simulink model "formationControl"  (R2021b)
settings: Solver=FixedStepAuto  StartTime=0.0  StopTime=20  FixedStep=0.01  RelTol=1e-3
values from neighbouring files (symbols this model uses):
  optimalPath = cat(1,optimalPath,invPathTemp)    [CompareBruteForce.m]    (also in main2.m; main3.m; main5.m; main6.m)
  startPoint1 = [currentX;currentY;atan2(optimalPath(i,2)+.5-currentY,optimalPath(i,1)+.5-currentX)]    [main2.m]    (also in main3.m = [currentX1;currentY1;atan2(optimalPath(i,2)+.5-currentY1,opt; main5.m = [currentX1;currentY1;theta_x1]; main6.m = [currentX1;currentY1;atan2(optimalPath(i,2)+.5-currentY1,opt; main7.m = [currentX1;currentY1;theta_x1])
  startPoint2 = [currentX2;currentY2;currentTeta2]    [main3.m]    (also in main5.m; main6.m; main7.m; main8.m = [currentX2;currentY2;theta_x1])
  startPoint3 = [currentX3;currentY3;currentTeta3]    [main3.m]    (also in main5.m; main6.m; main7.m; main8.m = [currentX3;currentY3;theta_x1])
  targetPoint1 = [optimalPath(1,1)+.5,optimalPath(1,2)+.5]    [main2.m]    (also in main3.m; main5.m; main6.m; main7.m)
  theta = toDegree(x(3))    [CalcHeadingEval.m]    (also in DynamicWindowApproachSample.m; main3.m = atan2(dy,dx); main5.m = atan2(dy,dx); main6.m = atan2(dy,dx))
  v = 3    [mTSPandFormation.m]    (also in main3.m = sqrt(vx.^2+vy.^2); main5.m = sqrt(vx.^2+vy.^2); main6.m = sqrt(vx.^2+vy.^2); main7.m = sqrt(vx.^2+vy.^2))
  vw_dt = [0.04;0]    [main3.m]    (also in main5.m; main6.m; main7.m; main8.m)
  w = edgew(p(j,k),p(j,k+1))    [CompareBruteForce.m]    (also in main3.m = dtheta ./ gradient(t_temp); main5.m = dtheta ./ gradient(t_temp); main6.m = dtheta ./ gradient(t_temp); main7.m = dtheta ./ gradient(t_temp))
settings Model: Creator=laptop  LastModifiedBy=SPKT2021
settings DataIOCC: ReturnWorkspaceOutputs=off

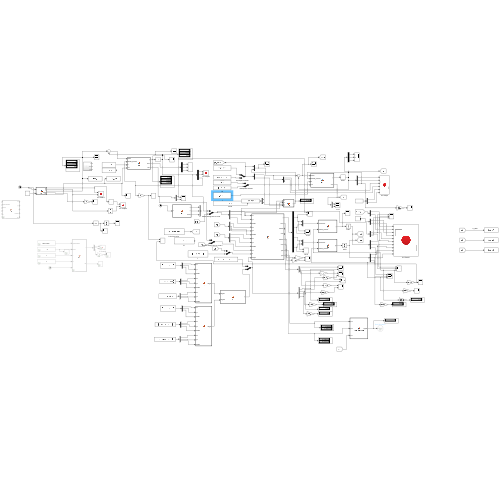
[thumbnail: Simulink's stored preview of the top-level diagram]
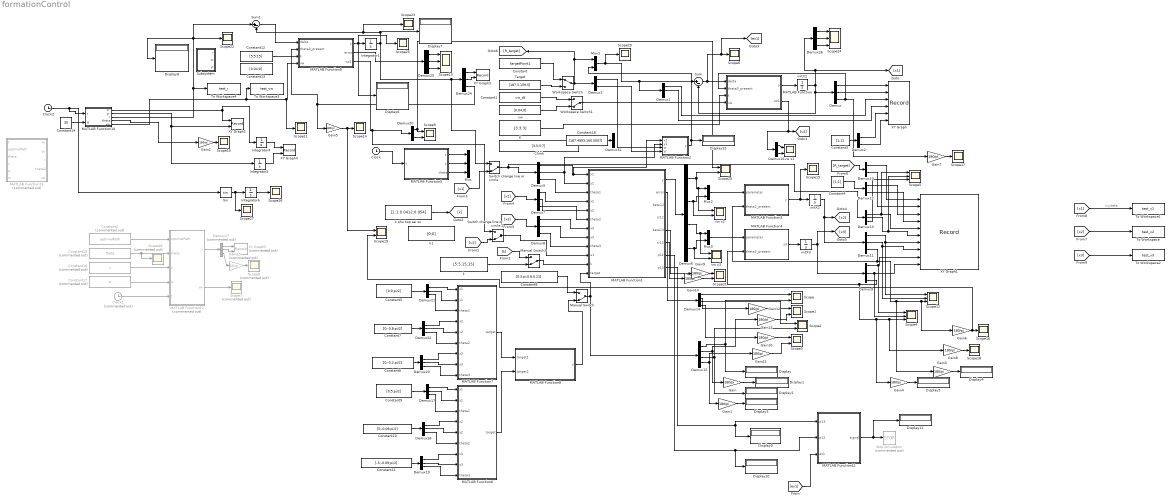
== system formationControl ==
  note: x;y;teta
  Chính : Constant  Value=[3.5;5;7]
  Clock : Clock
  Clock1 : Clock  Commented=on
  Clock2 : Clock
  Constant : Constant  Value=targetPoint1
  Constant1 : Constant  Value=vw_dt
  Constant10 : Constant  Value=[5;-0.09;pi/2]
  Constant11 : Constant  Value=[-5;-0.09;pi/2]
  Constant12 : Constant  Value=[5;5;15]
  Constant13 : Constant  Value=[0.04;0]
  Constant14 : Constant  Value=30
  Constant15 : Constant  Commented=on  Value=theta
  Constant16 : Constant  Commented=on  Value=v
  Constant17 : Constant  Commented=on  Value=w
  Constant18 : Constant  Value=[187.4993;160.5007]
  Constant2 : Constant  Commented=on  Value=optimalPath
  Constant3 : Constant  Value=[1;1]
  Constant4 : Constant  Value=[1;1]
  Constant5 : Constant  Value=[0;0;pi/2]
  Constant6 : Constant  Value=[0;-0.2;pi/2]
  Constant7 : Constant  Value=[0;-0.8;pi/2]
  Constant8 : Constant  Value=[0.3;pi;0.6;0.21]
  Constant9 : Constant  Value=[0;5;pi/2]
  Demux{,1,5,7..9,11,13,17..19,21..26} (17 alike) : Demux  Outputs=3
  Demux{2..3,10,12,16,20,31} (7 alike) : Demux  Outputs=2
  Demux14 : Demux
  Demux15 : Demux
  Demux27 : Demux  Commented=on  Outputs=3
  Demux6 : Demux
  Display{,1..12} (13 alike) : Display
  Gain{,1..14} (15 alike) : Gain  Gain=180/pi
  Gain15 : Gain  Commented=on  Gain=180/pi
  Integrator1 : Integrator  InitialCondition=[3;0;pi/2]
  Integrator4 : Integrator  InitialCondition=[0;0]
  Integrator5 : Integrator  InitialCondition=[0;0]
  Integrator6 : Integrator  InitialCondition=[0;0]
  K : Constant  Value=[3;3;3]
  MATLAB Function : MATLAB Function  TreatAsAtomicUnit=on
  MATLAB Function1 : MATLAB Function  TreatAsAtomicUnit=on
  MATLAB Function10 : MATLAB Function  TreatAsAtomicUnit=on
  MATLAB Function11 : MATLAB Function  TreatAsAtomicUnit=on
  MATLAB Function12 : MATLAB Function  Commented=on  TreatAsAtomicUnit=on
  MATLAB Function13 : MATLAB Function  Commented=on  TreatAsAtomicUnit=on
  MATLAB Function2 : MATLAB Function  TreatAsAtomicUnit=on
  MATLAB Function3 : MATLAB Function  TreatAsAtomicUnit=on
  MATLAB Function4 : MATLAB Function  TreatAsAtomicUnit=on
  MATLAB Function5 : MATLAB Function  TreatAsAtomicUnit=on
  MATLAB Function6 : MATLAB Function  TreatAsAtomicUnit=on
  MATLAB Function7 : MATLAB Function  TreatAsAtomicUnit=on
  MATLAB Function8 : MATLAB Function  TreatAsAtomicUnit=on
  MATLAB Function9 : MATLAB Function  TreatAsAtomicUnit=on
  Manual Switch : ManualSwitch  CurrentSetting=0
  Manual Switch3 : ManualSwitch  CurrentSetting=0
  Mux : Mux  Inputs=3
  Mux1 : Mux  Inputs=2
  Mux2 : Mux  Inputs=2
  Mux3 : Mux  Inputs=2
  Scope{,1..3,9,19..21} (8 alike) : Scope  NumInputPorts=2
  Scope{6,10..11,14..18,22..23,25..27,29} (14 alike) : Scope
  Scope{4..5,12..13,24} (5 alike) : Scope  NumInputPorts=3
  Scope28 : Scope  Commented=on
  Scope7 : Scope  Commented=on
  Scope8 : Scope  Commented=on
  Sin : Trigonometry
  Stop Simulation : Stop  Commented=on
  Subsystem : Subsystem
  Sum : Sum  Inputs=|+-
  Sum1 : Sum  Inputs=|+-
  Switch change line or circle : ManualSwitch  CurrentSetting=0
  Switch change line or circle 2 : ManualSwitch  CurrentSetting=0
  Target : Constant  Value=[187.5,159.5]
  To Workspace : ToWorkspace  VariableName=test_x2  SampleTime=-1
  To Workspace1 : ToWorkspace  VariableName=test_x1  SampleTime=-1
  To Workspace2 : ToWorkspace  VariableName=test_x3  SampleTime=-1
  To Workspace3 : ToWorkspace  VariableName=test_vw  SampleTime=-1
  To Workspace4 : ToWorkspace  VariableName=test_r  SampleTime=-1
  Workspace Switch : ManualSwitch
  Workspace Switch1 : ManualSwitch  CurrentSetting=0
  XY Graph : Record  FileSettingsInternal="{\"entries\":[{\"content\":{\"excelSettings\":{\"content\":{},\"type\":\"Streamout.ExcelSettings\"}},\"type\":\"Streamout.FileSettingStorage\",\"uuid\":\"b5055ff0-990a-4c3a-b253-25ae7f3dcace\"}],\"packageUris\":[\"http://schema.mathworks.com/mf0/streamout_blocks/R2020a\"],\"version\":\"1.0\"}"  Layout=[1 1]  SignalsInternal="{\"entries\":[{\"content\":{\"signals\":[{\"content\":{\"blockPath\":[\"formationControl/XY Graph\"],\"channel\":[],\"dimensions\":[1],\"domain\":\"formationControl/XY Graph\",\"lineColor\":\"#a2142f\",\"plots\":[1],\"port\":1,\"sid\":[\"\"],\"signalID\":561968,\"signalName\":\"Demux:1\"},\"type\":\"RecordBlkView.Signal\",\"uuid\":\"e63b4134-e2ed-49bd-bde4-29753b3ad62d\"},{\"content\":{\"blockPath\":[\"formationControl/XY Graph\"],\"channel\":[],\"dimensions\":[1],\"domain\":\"formationControl/XY Graph\",\"lineColor\":\"#139fff\",\"plots\":[1],\"port\":2,\"sid\":[\"\"],\"signalID\":561972,\"signalName\":\"Demux:2\"},\"type\":\"RecordBlkView.Signal\",\"uuid\":\"707cade7-eafc-4262-9cee-70ee2dfbe21c\"},{\"content\":{\"blockPath\":[\"formationControl/XY Graph\"],\"channel\":[],\"dimensions\":[1],\"domain\":\"formationControl/XY Graph\",\"lineColor\":\"#0072bd\",\"plots\":[1],\"port\":3,\"sid\":[\"\"],\"signalID\":561976,\"signalName\":\"Demux1:1\"},\"type\":\"RecordBlkView.Signal\",\"uuid\":\"0a2b94da-b4de-41ed-a62f-eca595da52b7\"},{\"content\":{\"blockPath\":[\"formationControl/XY Graph\"],\"channel\":[],\"dimensions\":[1],\"domain\":\"formationControl/XY Graph\",\"lineColor\":\"#d95319\",\"plots\":[1],\"port\":4,\"sid\":[\"\"],\"signalID\":561980,\"signalName\":\"Demux1:2\"},\"type\":\"RecordBlkView.Signal\",\"uuid\":\"faace5d8-a62c-4b29-bb0e-d2e558786eb1\"},{\"content\":{\"blockPath\":[\"formationControl/XY Graph\"],\"channel\":[],\"dimensions\":[1],\"domain\":\"formationControl/XY Graph\",\"lineColor\":\"#edb120\",\"plots\":[],\"port\":5,\"sid\":[\"\"],\"signalID\":562042,\"signalName\":\"Demux2:1\"},\"type\":\"RecordBlkView.Signal\",\"uuid\":\"74eace78-24eb-4fdf-b1d5-15840ce82639\"},{\"content\":{\"blockPath\":[\"formationControl/XY Graph\"],\"channel\":[],\"dimensions\":[1],\"domain\":\"formationControl/XY Graph\",\"lineColor\":\"#7e2f8e\",\"plots\":[],\"port\":6,\"sid\":[\"\"],\"signalID\":562046,\"signalName\":\"Demux2:2\"},\"type\":\"RecordBlkView.Signal\",\"uuid\":\"791b3ccc-bb9e-4ae3-a063-47e8357b569f\"}]},\"type\":\"RecordBlkView.InputSignals\",\"uuid\":\"a397a2d8-c02c-4be2-99ce-39e8efd3ceb2\"}],\"packageUris\":[\"http://schema.mathworks.com/mf0/streamout_blocks/R2020a\"],\"version\":\"1.0\"}"  VisualizationBindings="{\"xyplotplugin\":{\"info\":[{\"series\":[{\"bindingParametersList\":[{\"parameter\":\"Y-Axis\",\"signalID\":561980,\"signalName\":\"Demux1:2\"},{\"parameter\":\"X-Axis\",\"signalID\":561976,\"signalName\":\"Demux1:1\"}],\"seriesID\":8361},{\"bindingParametersList\":[{\"parameter\":\"Y-Axis\",\"signalID\":561972,\"signalName\":\"Demux:2\"},{\"parameter\":\"X-Axis\",\"signalID\":561968,\"signalName\":\"Demux:1\"}],\"seriesID\":45845}],\"subplotID\":1},{\"series\":[],\"subplotID\":2}]}}"  CompatibilityTag=XY
  XY Graph1 : Record  FileSettingsInternal="{\"entries\":[{\"content\":{\"excelSettings\":{\"content\":{},\"type\":\"Streamout.ExcelSettings\"}},\"type\":\"Streamout.FileSettingStorage\",\"uuid\":\"f4eddb40-bf7c-43c4-9250-d6d81d750d9e\"}],\"packageUris\":[\"http://schema.mathworks.com/mf0/streamout_blocks/R2020a\"],\"version\":\"1.0\"}"  Layout=[1 1]  SignalsInternal="{\"entries\":[{\"content\":{\"signals\":[{\"content\":{\"blockPath\":[\"formationControl/XY Graph1\"],\"channel\":[],\"dimensions\":[1],\"domain\":\"formationControl/XY Graph1\",\"lineColor\":\"#a2142f\",\"plots\":[],\"port\":1,\"sid\":[\"\"],\"signalID\":561984,\"signalName\":\"Demux10:1\"},\"type\":\"RecordBlkView.Signal\",\"uuid\":\"8c3099c7-507a-43dc-9679-003c8e2b0fad\"},{\"content\":{\"blockPath\":[\"formationControl/XY Graph1\"],\"channel\":[],\"dimensions\":[1],\"domain\":\"formationControl/XY Graph1\",\"lineColor\":\"#139fff\",\"plots\":[],\"port\":2,\"sid\":[\"\"],\"signalID\":561988,\"signalName\":\"Demux10:2\"},\"type\":\"RecordBlkView.Signal\",\"uuid\":\"c0ce0b80-6bff-4357-a116-862bc05278e8\"},{\"content\":{\"blockPath\":[\"formationControl/XY Graph1\"],\"channel\":[],\"dimensions\":[1,1],\"domain\":\"formationControl/XY Graph1\",\"lineColor\":\"#64d413\",\"plots\":[1],\"port\":5,\"sid\":[\"\"],\"signalID\":561992,\"signalName\":\"Demux13:1\"},\"type\":\"RecordBlkView.Signal\",\"uuid\":\"0fa45c33-8d0f-4364-9dfd-7943371a5639\"},{\"content\":{\"blockPath\":[\"formationControl/XY Graph1\"],\"channel\":[],\"dimensions\":[1,1],\"domain\":\"formationControl/XY Graph1\",\"lineColor\":\"#ff13a6\",\"plots\":[1],\"port\":6,\"sid\":[\"\"],\"signalID\":561996,\"signalName\":\"Demux13:2\"},\"type\":\"RecordBlkView.Signal\",\"uuid\":\"f72f9b85-cbc4-4606-ad4e-4a800cefdb27\"},{\"content\":{\"blockPath\":[\"formationControl/XY Graph1\"],\"channel\":[],\"dimensions\":[1,1],\"domain\":\"formationControl/XY Graph1\",\"lineColor\":\"#fe330a\",\"plots\":[1],\"port\":7,\"sid\":[\"\"],\"signalID\":562000,\"signalName\":\"Demux11:1\"},\"type\":\"RecordBlkView.Signal\",\"uuid\":\"1e6c43bc-44ba-4aff-8d4e-9963f198e577\"},{\"content\":{\"blockPath\":[\"formationControl/XY Graph1\"],\"channel\":[],\"dimensions\":[1,1],\"domain\":\"formationControl/XY Graph1\",\"lineColor\":\"#22b573\",\"plots\":[1],\"port\":8,\"sid\":[\"\"],\"signalID\":562004,\"signalName\":\"Demux11:2\"},\"type\":\"RecordBlkView.Signal\",\"uuid\":\"02b03434-467e-4bcb-89ce-f3374234228c\"},{\"content\":{\"blockPath\":[\"formationControl/XY Graph1\"],\"channel\":[],\"dimensions\":[1,1],\"domain\":\"formationControl/XY Graph1\",\"lineColor\":\"#a2142f\",\"plots\":[1],\"port\":9,\"sid\":[\"\"],\"signalID\":562008,\"signalName\":\"Demux9:1\"},\"type\":\"RecordBlkView.Signal\",\"uuid\":\"73795ee3-c77a-4222-9da6-29a7e69df84b\"},{\"content\":{\"blockPath\":[\"formationControl/XY Graph1\"],\"channel\":[],\"dimensions\":[1,1],\"domain\":\"formationControl/XY Graph1\",\"lineColor\":\"#139fff\",\"plots\":[1],\"port\":10,\"sid\":[\"\"],\"signalID\":562012,\"signalName\":\"Demux9:2\"},\"type\":\"RecordBlkView.Signal\",\"uuid\":\"98f6643e-ac09-4f18-9082-ac15710b3409\"},{\"content\":{\"blockPath\":[\"formationControl/XY Graph1\"],\"channel\":[],\"dimensions\":[1],\"domain\":\"formationControl/XY Graph1\",\"lineColor\":\"#ff6929\",\"plots\":[],\"port\":3,\"sid\":[\"\"],\"signalID\":562050,\"signalName\":\"Demux12:1\"},\"type\":\"RecordBlkView.Signal\",\"uuid\":\"600281dc-aa09-4b58-ac4f-40cdebe3cee6\"},{\"content\":{\"blockPath\":[\"formationControl/XY Graph1\"],\"channel\":[],\"dimensions\":[1],\"domain\":\"formationControl/XY Graph1\",\"lineColor\":\"#b746ff\",\"plots\":[],\"port\":4,\"sid\":[\"\"],\"signalID\":562054,\"signalName\":\"Demux12:2\"},\"type\":\"RecordBlkView.Signal\",\"uuid\":\"17bb4773-f403-4cec-b4d0-29764e3cdb02\"}]},\"type\":\"RecordBlkView.InputSignals\",\"uuid\":\"fc6bf10a-84a8-427f-b839-36d29293a552\"}],\"packageUris\":[\"http://schema.mathworks.com/mf0/streamout_blocks/R2020a\"],\"version\":\"1.0\"}"  VisualizationBindings="{\"xyplotplugin\":{\"info\":[{\"series\":[{\"bindingParametersList\":[{\"parameter\":\"Y-Axis\",\"signalID\":562012,\"signalName\":\"Demux9:2\"},{\"parameter\":\"X-Axis\",\"signalID\":562008,\"signalName\":\"Demux9:1\"}],\"seriesID\":25155},{\"bindingParametersList\":[{\"parameter\":\"X-Axis\",\"signalID\":561992,\"signalName\":\"Demux13:1\"},{\"parameter\":\"Y-Axis\",\"signalID\":561996,\"signalName\":\"Demux13:2\"}],\"seriesID\":16221},{\"bindingParametersList\":[{\"parameter\":\"X-Axis\",\"signalID\":562000,\"signalName\":\"Demux11:1\"},{\"parameter\":\"Y-Axis\",\"signalID\":562004,\"signalName\":\"Demux11:2\"}],\"seriesID\":6192}],\"subplotID\":1},{\"series\":[],\"subplotID\":2},{\"series\":[],\"subplotID\":9},{\"series\":[],\"subplotID\":10}]}}"  CompatibilityTag=XY
  XY Graph2 : Record  FileSettingsInternal="{\"entries\":[{\"content\":{\"excelSettings\":{\"content\":{},\"type\":\"Streamout.ExcelSettings\"}},\"type\":\"Streamout.FileSettingStorage\",\"uuid\":\"bbd09a98-5208-4554-9354-024d8c7fe0b6\"}],\"packageUris\":[\"http://schema.mathworks.com/mf0/streamout_blocks/R2020a\"],\"version\":\"1.0\"}"  Layout=[1 1]  SignalsInternal="{\"entries\":[{\"content\":{\"signals\":[{\"content\":{\"blockPath\":[\"formationControl/XY Graph2\"],\"channel\":[],\"dimensions\":[1],\"domain\":\"formationControl/XY Graph2\",\"lineColor\":\"#0072bd\",\"plots\":[1],\"port\":1,\"sid\":[\"\"],\"signalID\":562016,\"signalName\":\"MATLAB Function10:1\"},\"type\":\"RecordBlkView.Signal\",\"uuid\":\"aba93bcb-ead4-4577-b090-7f5bc0fcbf51\"},{\"content\":{\"blockPath\":[\"formationControl/XY Graph2\"],\"channel\":[],\"dimensions\":[1],\"domain\":\"formationControl/XY Graph2\",\"lineColor\":\"#d95319\",\"plots\":[1],\"port\":2,\"sid\":[\"\"],\"signalID\":562020,\"signalName\":\"MATLAB Function10:2\"},\"type\":\"RecordBlkView.Signal\",\"uuid\":\"7b760fd5-6f6b-42c4-a1b4-18eec4e19632\"}]},\"type\":\"RecordBlkView.InputSignals\",\"uuid\":\"af8d5546-1592-4a3c-bd27-597adbd4dc42\"}],\"packageUris\":[\"http://schema.mathworks.com/mf0/streamout_blocks/R2020a\"],\"version\":\"1.0\"}"  VisualizationBindings="{\"xyplotplugin\":{\"info\":[{\"series\":[{\"bindingParametersList\":[{\"parameter\":\"X-Axis\",\"signalID\":562016,\"signalName\":\"MATLAB Function10:1\"},{\"parameter\":\"Y-Axis\",\"signalID\":562020,\"signalName\":\"MATLAB Function10:2\"}],\"seriesID\":32060}],\"subplotID\":1}]}}"  CompatibilityTag=XY
  XY Graph3 : Record  FileSettingsInternal="{\"entries\":[{\"content\":{\"excelSettings\":{\"content\":{},\"type\":\"Streamout.ExcelSettings\"}},\"type\":\"Streamout.FileSettingStorage\",\"uuid\":\"17b369dc-59dc-4738-87bd-0ae67a1d530c\"}],\"packageUris\":[\"http://schema.mathworks.com/mf0/streamout_blocks/R2020a\"],\"version\":\"1.0\"}"  Layout=[1 1]  SignalsInternal="{\"entries\":[{\"content\":{\"signals\":[{\"content\":{\"blockPath\":[\"formationControl/XY Graph3\"],\"channel\":[],\"dimensions\":[1,1],\"domain\":\"formationControl/XY Graph3\",\"lineColor\":\"#0072bd\",\"plots\":[1],\"port\":1,\"sid\":[\"\"],\"signalID\":562024,\"signalName\":\"Demux24:1\"},\"type\":\"RecordBlkView.Signal\",\"uuid\":\"48614805-dc79-436c-ab69-2c2dfbf3428a\"},{\"content\":{\"blockPath\":[\"formationControl/XY Graph3\"],\"channel\":[],\"dimensions\":[1,1],\"domain\":\"formationControl/XY Graph3\",\"lineColor\":\"#d95319\",\"plots\":[1],\"port\":2,\"sid\":[\"\"],\"signalID\":562028,\"signalName\":\"Demux24:2\"},\"type\":\"RecordBlkView.Signal\",\"uuid\":\"5ef9c048-c3da-4d3a-81e6-ba00ac53b929\"}]},\"type\":\"RecordBlkView.InputSignals\",\"uuid\":\"9ef3bded-a44e-4d83-9b31-ae2182672258\"}],\"packageUris\":[\"http://schema.mathworks.com/mf0/streamout_blocks/R2020a\"],\"version\":\"1.0\"}"  VisualizationBindings="{\"xyplotplugin\":{\"info\":[{\"series\":[{\"bindingParametersList\":[{\"parameter\":\"X-Axis\",\"signalID\":562024,\"signalName\":\"Demux24:1\"},{\"parameter\":\"Y-Axis\",\"signalID\":562028,\"signalName\":\"Demux24:2\"}],\"seriesID\":56942}],\"subplotID\":1}]}}"  CompatibilityTag=XY
  XY Graph4 : Record  FileSettingsInternal="{\"entries\":[{\"content\":{\"excelSettings\":{\"content\":{},\"type\":\"Streamout.ExcelSettings\"}},\"type\":\"Streamout.FileSettingStorage\",\"uuid\":\"eee1474c-db82-48e3-be20-d8be3a7b9364\"}],\"packageUris\":[\"http://schema.mathworks.com/mf0/streamout_blocks/R2020a\"],\"version\":\"1.0\"}"  Layout=[1 1]  SignalsInternal="{\"entries\":[{\"content\":{\"signals\":[{\"content\":{\"blockPath\":[\"formationControl/XY Graph4\"],\"channel\":[],\"dimensions\":[2],\"domain\":\"formationControl/XY Graph4\",\"hasChildren\":true,\"lineColor\":\"#ff6929\",\"plots\":[],\"port\":1,\"sid\":[\"\"],\"signalID\":562032,\"signalName\":\"Integrator4\"},\"type\":\"RecordBlkView.Signal\",\"uuid\":\"9ee344e4-1d26-45a8-ba78-b3c0b50b027a\"},{\"content\":{\"blockPath\":[\"formationControl/XY Graph4\"],\"channel\":[1],\"dimensions\":[2],\"domain\":\"formationControl/XY Graph4\",\"lineColor\":\"#ff13a6\",\"parentID\":562032,\"plots\":[1],\"port\":1,\"sid\":[\"\"],\"signalID\":562033,\"signalName\":\"Integrator4\"},\"type\":\"RecordBlkView.Signal\",\"uuid\":\"2c4e1fb2-3731-44d4-a969-a9bd2b90733b\"},{\"content\":{\"blockPath\":[\"formationControl/XY Graph4\"],\"channel\":[],\"dimensions\":[2],\"domain\":\"formationControl/XY Graph4\",\"hasChildren\":true,\"lineColor\":\"#64d413\",\"plots\":[],\"port\":2,\"sid\":[\"\"],\"signalID\":562037,\"signalName\":\"Integrator5\"},\"type\":\"RecordBlkView.Signal\",\"uuid\":\"afac8585-8249-41c7-8222-482c13fc86ec\"},{\"content\":{\"blockPath\":[\"formationControl/XY Graph4\"],\"channel\":[1],\"dimensions\":[2],\"domain\":\"formationControl/XY Graph4\",\"lineColor\":\"#22b573\",\"parentID\":562037,\"plots\":[],\"port\":2,\"sid\":[\"\"],\"signalID\":562038,\"signalName\":\"Integrator5\"},\"type\":\"RecordBlkView.Signal\",\"uuid\":\"17174f1f-37b5-4fe6-a897-6887e4f5ae3c\"},{\"content\":{\"blockPath\":[\"formationControl/XY Graph4\"],\"channel\":[2],\"dimensions\":[2],\"domain\":\"formationControl/XY Graph4\",\"lineColor\":\"#ff6929\",\"parentID\":562032,\"plots\":[1],\"port\":1,\"sid\":[\"\"],\"signalID\":562058,\"signalName\":\"Integrator4\"},\"type\":\"RecordBlkView.Signal\",\"uuid\":\"643a3014-d775-4f6f-9dc6-3c6f2119b9c7\"},{\"content\":{\"blockPath\":[\"formationControl/XY Graph4\"],\"channel\":[2],\"dimensions\":[2],\"domain\":\"formationControl/XY Graph4\",\"lineColor\":\"#b746ff\",\"parentID\":562037,\"plots\":[],\"port\":2,\"sid\":[\"\"],\"signalID\":562059,\"signalName\":\"Integrator5\"},\"type\":\"RecordBlkView.Signal\",\"uuid\":\"4c220cfa-f8b1-4858-ba5c-4f74ffe338aa\"}]},\"type\":\"RecordBlkView.InputSignals\",\"uuid\":\"4427a746-86d7-4809-ba60-0aa2c1196432\"}],\"packageUris\":[\"http://schema.mathworks.com/mf0/streamout_blocks/R2020a\"],\"version\":\"1.0\"}"  VisualizationBindings="{\"xyplotplugin\":{\"info\":[{\"series\":[{\"bindingParametersList\":[{\"parameter\":\"X-Axis\",\"signalID\":562033,\"signalName\":\"Integrator4(1)\"},{\"parameter\":\"Y-Axis\",\"signalID\":562058,\"signalName\":\"Integrator4(2)\"}],\"seriesID\":36027}],\"subplotID\":1}]}}"  CompatibilityTag=XY
  XY Graph5 : Record  Commented=on  FileSettingsInternal="{\"entries\":[{\"content\":{\"excelSettings\":{\"content\":{},\"type\":\"Streamout.ExcelSettings\"}},\"type\":\"Streamout.FileSettingStorage\",\"uuid\":\"2d92b61e-650a-40c4-a1c8-d9bbc27f0ede\"}],\"packageUris\":[\"http://schema.mathworks.com/mf0/streamout_blocks/R2020a\"],\"version\":\"1.0\"}"  Layout=[1 1]  SignalsInternal="{\"entries\":[{\"content\":{\"signals\":[{\"content\":{\"blockPath\":[\"formationControl/XY Graph5\"],\"channel\":[],\"dimensions\":[1],\"domain\":\"formationControl/XY Graph5\",\"lineColor\":\"#edb120\",\"plots\":[],\"port\":1,\"sid\":[],\"signalID\":257,\"signalName\":\"Demux27:1\"},\"type\":\"RecordBlkView.Signal\",\"uuid\":\"ef02fb2f-8446-4abe-973e-69e80fa250d6\"},{\"content\":{\"blockPath\":[\"formationControl/XY Graph5\"],\"channel\":[],\"dimensions\":[1],\"domain\":\"formationControl/XY Graph5\",\"lineColor\":\"#7e2f8e\",\"plots\":[],\"port\":2,\"sid\":[],\"signalID\":260,\"signalName\":\"Demux27:2\"},\"type\":\"RecordBlkView.Signal\",\"uuid\":\"8fae97be-fc71-4d0b-906e-0cb1667f536b\"}]},\"type\":\"RecordBlkView.InputSignals\",\"uuid\":\"41859449-d739-4903-a015-30797226d830\"}],\"packageUris\":[\"http://schema.mathworks.com/mf0/streamout_blocks/R2020a\"],\"version\":\"1.0\"}"  VisualizationBindings="{\"xyplotplugin\":{\"info\":[{\"series\":[],\"subplotID\":1}]}}"  CompatibilityTag=XY
  initX1 : Integrator  InitialCondition=startPoint1
  initX2 : Integrator  InitialCondition=startPoint2
  initX3 : Integrator  InitialCondition=startPoint3
  k : Constant  Value=[5;5;15;15]
  k phu hop sai so : Constant  Value=[1;1;0.0412;0.054]
  k1 : Constant  Value=[0;0]
  vw : Constant  Value=[0.04;0]
  vw x1 : Scope  NumInputPorts=2
  vw x2 : Scope  NumInputPorts=2
  vw x3 : Scope  NumInputPorts=2
  wires:
  Demux12/2 -> XY Graph1/4
  Demux5/1 -> MATLAB Function2/1(x1), MATLAB Function1/1(x1)
  Demux/1 -> XY Graph/1
  MATLAB Function5/2(y) -> Mux/2
  Gain/1 -> Display1/1
  Demux11/2 -> Scope12/2, XY Graph1/8
  Demux14/3 -> Scope2/1
  Demux7/3 -> MATLAB Function1/6(theta2)
  Demux9/1 -> Scope4/1, XY Graph1/9
  MATLAB Function5/3(theta) -> Mux/3
  Demux1/2 -> XY Graph/4
  Clock/1 -> MATLAB Function5/1(t)
  k phu hop sai so/1 -> [k]
  MATLAB Function3/1(y) -> Scope15/1, initX2/1
  Demux16/2 -> vw x1/2
  Demux8/1 -> MATLAB Function1/7(x3)
  Demux16/1 -> vw x1/1
  Demux21/1 -> MATLAB Function7/1(x1)
  Demux9/2 -> Scope4/2, XY Graph1/10
  Sum/1 -> [ex1], Scope6/1, MATLAB Function/1(delta)
  MATLAB Function5/1(x) -> Mux/1
  Demux/2 -> XY Graph/2
  MATLAB Function1/2(error) -> Demux14/1
  Demux22/2 -> MATLAB Function7/5(y2)
  Mux1/1 -> Scope29/1, Sum/1, Demux1/1
  Demux2/2 -> XY Graph/6
  Demux1/1 -> XY Graph/3
  Demux21/2 -> MATLAB Function7/2(y1)
  Demux10/2 -> XY Graph1/2
  MATLAB Function/1(y) -> initX1/1
  [x3] -> Demux8/1
  Demux8/2 -> MATLAB Function1/8(y3)
  Demux15/1 -> Scope/2, Display/1
  Demux6/2 -> vw x2/2, Mux2/2
  Demux2/1 -> XY Graph/5
  Demux6/1 -> Scope20/2, vw x2/1, Mux2/1
  Demux10/1 -> XY Graph1/1
  MATLAB Function/2(vw1) -> Demux16/1, [u1]
  Demux13/1 -> Scope5/1, XY Graph1/5
  Demux14/2 -> Gain12/1
  Demux11/1 -> Scope12/1, XY Graph1/7
  Demux5/3 -> MATLAB Function1/3(theta1)
  initX2/1 -> Demux11/1, [x2]
  Demux14/4 -> Gain10/1
  Demux5/2 -> MATLAB Function1/2(y1), MATLAB Function2/2(y1)
  [x2] -> Demux7/1
  Demux15/2 -> Gain13/1, Gain/1
  Constant3/1 -> Demux2/1
  Demux8/3 -> MATLAB Function1/9(theta3)
  Demux7/2 -> MATLAB Function1/5(y2)
  Demux7/1 -> MATLAB Function1/4(x2)
  Demux13/2 -> Scope5/2, XY Graph1/6
  [R_target] -> Demux10/1
  Demux23/1 -> MATLAB Function7/7(x3)
  Demux6/4 -> vw x3/2, Mux3/2
  Mux2/1 -> MATLAB Function3/1(parameter)
  Demux15/3 -> Scope2/2, Display2/1
  Constant4/1 -> Demux12/1
  MATLAB Function4/1(y3) -> initX3/1
  Demux22/1 -> MATLAB Function7/4(x2)
  K/1 -> MATLAB Function/3(k)
  Manual Switch/1 -> MATLAB Function1/12(target), Demux15/1
  Constant8/1 -> Manual Switch/1
  Constant5/1 -> Demux21/1
  Demux15/4 -> Gain11/1, Gain1/1
  MATLAB Function1/1(y) -> Demux6/1
  initX3/1 -> [x3], Demux9/1
  Demux23/2 -> MATLAB Function7/8(y3)
  Demux14/1 -> Scope/1
  Demux22/3 -> MATLAB Function7/6(theta2)
  Demux12/1 -> XY Graph1/3
  initX1/1 -> Sum/2, Demux/1, Demux26/1, [x1]
  Demux21/3 -> MATLAB Function7/3(theta1)
  Demux23/3 -> MATLAB Function7/9(theta3)
  Demux19/3 -> MATLAB Function6/9(theta3)
  Demux17/3 -> MATLAB Function6/3(theta1)
  Demux18/3 -> MATLAB Function6/6(theta2)
  Demux19/2 -> MATLAB Function6/8(y3)
  Constant9/1 -> Demux17/1
  Demux18/1 -> MATLAB Function6/4(x2)
  Constant10/1 -> Demux18/1
  Demux19/1 -> MATLAB Function6/7(x3)
  MATLAB Function6/1(target) -> MATLAB Function8/2(target2)
  Demux17/2 -> MATLAB Function6/2(y1)
  Demux18/2 -> MATLAB Function6/5(y2)
  Demux17/1 -> MATLAB Function6/1(x1)
  Constant11/1 -> Demux19/1
  MATLAB Function7/1(target) -> MATLAB Function8/1(target1)
  MATLAB Function8/1(y) -> Manual Switch/2
  Demux6/3 -> vw x3/1, Mux3/1
  Gain1/1 -> Display3/1
  Constant6/1 -> Demux23/1
  Constant7/1 -> Demux22/1
  Integrator1/1 -> Display7/1, Scope23/1, Sum1/2, Switch change line or circle/1, Demux24/1
  Demux20/2 -> Scope9/2
  MATLAB Function9/3(vw1) -> Switch change line or circle 2/1, Demux20/1
  Demux20/1 -> Scope20/1, Scope9/1
  Gain2/1 -> Scope10/1
  Constant14/1 -> MATLAB Function10/2(tf)
  Constant12/1 -> MATLAB Function9/3(k)
  Clock2/1 -> Sin/1, MATLAB Function10/1(t)
  MATLAB Function9/1(y) -> Display6/1, Scope25/1, Integrator1/1
  Sum1/1 -> MATLAB Function9/1(delta)
  Demux13/3 -> Scope5/3
  Switch change line or circle/1 -> Demux13/1, Demux5/1
  [x1] -> Switch change line or circle/2
  Switch change line or circle 2/1 -> MATLAB Function1/10(u1)
  [u1] -> Switch change line or circle 2/2
  Gain3/1 -> Display4/1
  Gain4/1 -> Display5/1
  Manual Switch3/1 -> MATLAB Function1/11(k)
  [k] -> Manual Switch3/1
  k/1 -> Manual Switch3/2
  Demux24/3 -> MATLAB Function9/2(theta0_present), Gain5/1
  Demux25/1 -> Scope13/1
  Demux25/2 -> Scope13/2
  Demux25/3 -> Scope13/3
  MATLAB Function9/2(error) -> Demux25/1
  Demux11/3 -> MATLAB Function3/2(theta2_present), Gain3/1, Gain6/1, Scope12/3
  Gain6/1 -> Scope19/2, Scope16/1
  Gain7/1 -> Scope17/1
  Demux/3 -> Gain7/1, MATLAB Function/2(theta0_present)
  Demux24/1 -> XY Graph3/1
  Demux24/2 -> XY Graph3/2
  Gain8/1 -> Scope18/1
  Demux9/3 -> Gain4/1, Gain8/1, Scope4/3, MATLAB Function4/2(theta3_present)
  Gain10/1 -> Scope3/1
  Gain11/1 -> Scope3/2
  Gain12/1 -> Scope1/1
  Gain13/1 -> Scope1/2
  Gain5/1 -> Scope19/1, Scope14/1
  Gain9/1 -> Scope21/1
  Gain14/1 -> Scope21/2
  Demux26/1 -> Scope24/1
  Demux26/2 -> Scope24/2
  Demux26/3 -> Scope24/3
  MATLAB Function1/6(si13) -> Gain14/1
  MATLAB Function1/5(beta13) -> Gain9/1
  Mux3/1 -> MATLAB Function4/1(parameter)
  Integrator4/1 -> XY Graph4/1
  Integrator5/1 -> XY Graph4/2
  Sin/1 -> Scope27/1, Integrator6/1
  Integrator6/1 -> Scope26/1
  [x2] -> To Workspace/1
  [x1] -> To Workspace1/1
  [x3] -> To Workspace2/1
  Target/1 -> Workspace Switch/2
  Workspace Switch/1 -> Mux1/1, [R_target], Demux3/1
  Constant/1 -> Workspace Switch/1
  Workspace Switch1/1 -> MATLAB Function/4(vw)
  vw/1 -> Workspace Switch1/2
  Constant1/1 -> Workspace Switch1/1
  MATLAB Function11/1(signal) -> Display11/1, Stop Simulation/1
  MATLAB Function1/8(p13) -> Display9/1, MATLAB Function11/1(p13)
  MATLAB Function1/7(p12) -> Display10/1, MATLAB Function11/2(p12)
  [ex1] -> MATLAB Function11/3(ex1)
  Constant15/1 -> Scope28/1, MATLAB Function12/2(theta)
  Constant16/1 -> MATLAB Function12/3(v)
  Constant17/1 -> MATLAB Function12/4(w)
  Clock1/1 -> MATLAB Function12/5(t)
  MATLAB Function12/1(r) -> Demux27/1
  Demux27/1 -> XY Graph5/1
  Demux27/2 -> XY Graph5/2
  MATLAB Function12/2(vw) -> Scope7/1
  Gain15/1 -> Scope8/1
  Demux27/3 -> Gain15/1
  Constant2/1 -> MATLAB Function12/1(optimalPath)
  Constant18/1 -> Demux31/1
  Demux3/1 -> MATLAB Function2/3(xr)
  Demux3/2 -> MATLAB Function2/4(yr)
  MATLAB Function2/1(y) -> Mux1/2, Display12/1
  MATLAB Function10/1(xr) -> Integrator4/1, XY Graph2/1
  MATLAB Function10/2(yr) -> Integrator5/1, XY Graph2/2
  MATLAB Function10/3(r) -> Display8/1, Sum1/1, Scope22/1, To Workspace4/1
  MATLAB Function10/4(theta) -> Gain2/1
  MATLAB Function10/5(vw) -> To Workspace3/1, Scope11/1, MATLAB Function9/4(vw)

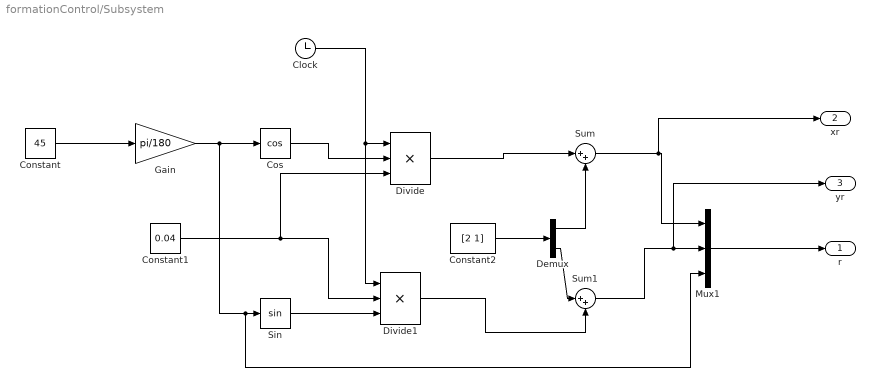
== system formationControl/Subsystem ==
  Clock : Clock
  Constant : Constant  Value=45
  Constant1 : Constant  Value=0.04
  Constant2 : Constant  Value=[2 1]
  Cos : Trigonometry  Operator=cos
  Demux : Demux  Outputs=2
  Divide : Product  Inputs=***
  Divide1 : Product  Inputs=***
  Gain : Gain  Gain=pi/180
  Mux1 : Mux  Inputs=3
  Sin : Trigonometry
  Sum : Sum  Inputs=|++
  Sum1 : Sum  Inputs=|++
  r : Outport
  xr : Outport  Port=2
  yr : Outport  Port=3
  wires:
  Cos/1 -> Divide/2
  Demux/2 -> Sum1/1
  Sin/1 -> Divide1/3
  Gain/1 -> Mux1/3, Sin/1, Cos/1
  Sum1/1 -> yr/1, Mux1/2
  Constant/1 -> Gain/1
  Constant1/1 -> Divide1/2, Divide/3
  Clock/1 -> Divide1/1, Divide/1
  Demux/1 -> Sum/2
  Divide/1 -> Sum/1
  Divide1/1 -> Sum1/2
  Sum/1 -> xr/1, Mux1/1
  Constant2/1 -> Demux/1
  Mux1/1 -> r/1

== matlab function formationControl/MATLAB Function8 ==
  data: target1 input; y output; target2 input
function y = fcn(target1, target2)
% if t<15
%     y = target1;
% else
%     y = target2;
% end
y = target2;

== matlab function formationControl/MATLAB Function10 ==
  data: t input; tf input; xr output; yr output; r output; theta output; vw output
function [xr,yr,r,theta,vw] = fcn(t,tf)
radius = 6;
omega = 2*pi/30;
v=omega*radius;

% xr = 5 + 4*cos(theta);
% yr = 5 + 4*sin(theta);

if t<tf
    theta =pi/2+ omega*t;
    xr =  radius*cos(theta - pi/2);
    yr = radius*sin(theta- pi/2);
else
    xr = radius*cos(2*pi);
    yr = radius*sin(2*pi);
    theta =pi/2+ omega*tf;
%     v=0;
%     omega=0;
end
r = [xr;yr;theta];
vw = [v;omega];

== matlab function formationControl/MATLAB Function9 ==
  data: delta input; y output; theta0_present input; k input; error output; vw input; vw1 output
function [y,error,vw1]= fcn(delta,theta0_present,k,vw)
A = [cos(theta0_present)   sin(theta0_present) 0;
       -sin(theta0_present) cos(theta0_present) 0;
         0                    0                    1];
e=A*delta;
v=vw(1);
w=vw(2);

V_c=[v*cos(e(3))+k(1)*e(1);
    w + k(2)*v*e(2) + k(3)*v*sin(e(3))];
Matrix = [cos(theta0_present) 0;
          sin(theta0_present) 0;
          0                   1];

% d=0.09;
% Matrix=[cos(theta0_present) -d*sin(theta0_present);
%         sin(theta0_present) d*cos(theta0_present);
%         0                   1];
u=Matrix*V_c;
y = u;
error = e;
vw1 = V_c;

== matlab function formationControl/MATLAB Function7 ==
  data: x1 input; target output; y1 input; theta1 input; x2 input; y2 input; theta2 input; x3 input; y3 input; theta3 input
function target = fcn(x1,y1,theta1,x2,y2,theta2,x3,y3,theta3)
%#codegen
d=0.09;
% 
% L12_x=x1-x2-d*cos(theta1);
% L12_y=y1-y2-d*sin(theta1);
% L13_x=x1-x3-d*cos(theta1);
% L13_y=y1-y3-d*sin(theta1);
% L23_x=x2-x3-d*cos(theta2);
% L23_y=y2-y3-d*sin(theta2);
L12_x=x1-x2-d*cos(theta2);
L12_y=y1-y2-d*sin(theta2);
L13_x=x1-x3-d*cos(theta3);
L13_y=y1-y3-d*sin(theta3);
L23_x=x2-x3-d*cos(theta3);
L23_y=y2-y3-d*sin(theta3);

L12=sqrt(L12_x^2+L12_y^2);
L13=sqrt(L13_x^2+L13_y^2);
L23=sqrt(L23_x^2+L23_y^2);

mega12=atan2(L12_y,L12_x)-theta1+pi;
if mega12<0
    k12=fix(-mega12/(2*pi));
    mega12 = 2*(k12+1)*pi +mega12;
end
mega13 = atan2(L13_y,L13_x)-theta1+pi;
if mega13<0 %khi mega <0 se xay ra hien tuong xoay tron
    k13=fix(-mega13/(2*pi));
    mega13 = 2*(k13+1)*pi +mega13;
end
mega23=atan2(L23_y,L23_x)-theta2+pi;
if mega23<0 %khi mega <0 se xay ra hien tuong xoay tron
    k23=fix(-mega23/(2*pi));
    mega23 = 2*(k23+1)*pi +mega23;
end
target=[L12;mega12;L13;mega13];

== matlab function formationControl/MATLAB Function11 ==
  data: p13 input; signal output; p12 input; ex1 input
function signal = stopSimulation(p13, p12, ex1)
if (p13(1) < 0.01)&&(p13(2) < 0.05)&&(p12(1) < 0.01)&&(p12(2) < 0.05)&&(ex1(1) < 0.0000001)&&(ex1(2) < 0.0000001)
    signal = 1;
else
    signal = 0;
end

== matlab function formationControl/MATLAB Function12 ==
  data: optimalPath input; r output; theta input; v input; w input; t input; vw output
function [r,vw] = fcn(optimalPath,theta,v,w,t)

if t*10<size(optimalPath,1)
    x = optimalPath(int16(t*10+1),1);
    y = optimalPath(int16(t*10+1),2);
    theta2 = theta(int16(t*10+1),1);
    v2 = v(int16(t*10+1),1);
    w2 = w(int16(t*10+1),1);
else
    x = optimalPath(end, 1);
    y = optimalPath(end, 2);
    theta2 = theta(end);
    v2 = v(end);
    w2 = w(end);
end
r = [x;y;theta2];
vw = [v2;w2];

== matlab function formationControl/MATLAB Function13 ==
  data: xx output; yy output; t input; optimalPath input; r output; theta2 output; theta input; v input; w input; m input; vw output
function [xx,yy,r,theta2,vw] = fcn(t,optimalPath,theta,v,w,m)
x = optimalPath(:,1).';
y = optimalPath(:,2).';
thetaSpline = theta.';
vSpline = v.';
wSpline = w.';

tt = linspace(0,1,m);
xx = spline(t, x, tt);
yy = spline(t, y, tt);
theta2 = spline(t, thetaSpline, tt);
vSpline2 = spline(t, vSpline, tt);
wSpline2 = spline(t, wSpline, tt);

r = [xx;yy;theta2];
vw = [vSpline2;wSpline2];

== matlab function formationControl/MATLAB Function1 ==
  data: x1 input; y output; y1 input; theta1 input; x2 input; y2 input; theta2 input; x3 input; y3 input; theta3 input; u1 input; k input; target input; error output; beta12 output; si12 output; beta13 output; si13 output; p12 output; p13 output
function [y,error,beta12,si12,beta13,si13,p12,p13] = fcn(x1,y1,theta1,x2,y2,theta2,x3,y3,theta3,u1,k,target)
%#coegen
if theta1<0
    k1=fix(-theta1/(2*pi));
    theta1 = 2*(k1+1)*pi +theta1;
end

d=0.09;
% L12_x=x1-x2-d*cos(theta1);
% L12_y=y1-y2-d*sin(theta1);
% L13_x=x1-x3-d*cos(theta1);
% L13_y=y1-y3-d*sin(theta1);
% L23_x=x2-x3-d*cos(theta2);
% L23_y=y2-y3-d*sin(theta2);
L12_x=x1-x2-d*cos(theta2);
L12_y=y1-y2-d*sin(theta2);
L13_x=x1-x3-d*cos(theta3);
L13_y=y1-y3-d*sin(theta3);
L23_x=x2-x3-d*cos(theta3);
L23_y=y2-y3-d*sin(theta3);

L12=sqrt(L12_x^2+L12_y^2);
L13=sqrt(L13_x^2+L13_y^2);
L23=sqrt(L23_x^2+L23_y^2);

mega12=atan2(L12_y,L12_x)-theta1+pi;
if mega12<0
    k12=fix(-mega12/(2*pi));
    mega12 = 2*(k12+1)*pi +mega12;
end
if mega12>(2*pi) %khi mega <0 se xay ra hien tuong xoay tron
    k12=fix(mega12/(2*pi));
    mega12 = mega12-2*(k12+1)*pi;
end
mega13=atan2(L13_y,L13_x)-theta1+pi;
if mega13<0 %khi mega <0 se xay ra hien tuong xoay tron
    k13=fix(-mega13/(2*pi));
    mega13 = 2*(k13+1)*pi +mega13;
end
if mega13>(2*pi) %khi mega <0 se xay ra hien tuong xoay tron
    k13=fix(mega13/(2*pi));
    mega13 = mega13-2*(k13+1)*pi;
end
mega23=atan2(L23_y,L23_x)-theta2+pi;


beta12=theta1-theta2;
beta13=theta1-theta3;
beta23=theta2-theta3;
% if beta12>pi
%     beta12 = pi;
% end
% if beta13>pi
%     beta13 = pi;
% end

si12=beta12+mega12;
si13=beta13+mega13;
si23=beta23+mega23;

% G2=[cos(si12)      d*sin(si12)     0         0;
%     -sin(si12)/L12 d*cos(si12)/L12 0         0;
%     0              0               cos(si13) d*sin(si13);
%     -cos(mega23)   0               cos(si23) d*sin(si23)];
% 
% F2=[-cos(mega12)     0;
%     sin(mega12)/L12 -1;
%     -cos(mega13)     0;
%     0                0];


% p= [k(1)*(target(1)-L12);
%     k(2)*(target(2)-mega12);
%     k(3)*(target(3)-L13);
%     k(4)*(target(4)-L23)];

G12=[cos(si12)      d*sin(si12);
    -sin(si12)/L12 d*cos(si12)/L12;
    ];

F12=[-cos(mega12)     0;
    sin(mega12)/L12  -1];

p12= [k(1)*(target(1)-L12);
    k(2)*(target(2)-mega12)];
%%%%%%
G13=[cos(si13)      d*sin(si13);
    -sin(si13)/L13 d*cos(si13)/L13];

F13=[-cos(mega13)     0;
    sin(mega13)/L13  -1];

p13= [k(1)*(target(3)-L13);
    k(2)*(target(4)-mega13)]; % neu de mega < 0 (-270do =90 do) thi khi tinh
                               %toan cos sin se khong anh huong nhung p3
                               %se bi sai so lon dan den w3 bị vọt lố dao động
% G23=[cos(si23)      d*sin(si23);
%     -sin(si23)/L23 d*cos(si23)/L23];
% 
% F23=[-cos(mega23)     0;
%     sin(mega23)/L23  -1];
% 
% p23= [k(1)*(target(5)-L23);
%     k(2)*(target(6)-mega23)]; % neu de mega < 0 (-270do =90 do) thi khi tinh
%                                %toan cos sin se khong anh huong nhung p3
%                                %se bi sai so lon dan den w3 bị vọt lố dao động
e=[L12;
mega12;
L13;
mega13];


u12=inv(G12)*(p12-F12*u1);
u13=inv(G13)*(p13-F13*u1);
limit=5;
if abs(u12(1)) >limit
    u12(1) =(u12(1)/abs(u12(1)))*limit;
end
if abs(u12(2))>limit
    u12(2) =(u12(2)/abs(u12(2)))*limit;
end
if abs(u13(1)) >limit
    u13(1) =(u13(1)/abs(u13(1)))*limit;
end
if abs(u13(2))>limit
    u13(2) =(u13(2)/abs(u13(2)))*limit;
end

u = [u12(1);u12(2);u13(1);u13(2)];
% u23=inv(G23)*(p23-F23*u1);
% u = [u12(1);u12(2);u23(1);u23(2)];
error=e;
y = u;
% c12=cos(si12)
% s12=sin(si12)
% v12=c12-s12
 
%  %%%%
% x4=1.35;
% y4 =2.0;
% theta4 = 2*pi/3;
% 
% L24_x=x2-x4-d*cos(theta4);
% L24_y=y2-y4-d*sin(theta4);
% 
% L24=sqrt(L24_x^2+L24_y^2);
% sita12 = theta1 - theta2 + mega12;
% sita24 = theta4 - theta2;
% 
% p4 = [k(1)*(target(1) - L12);
%       6*(0.1 - L24)];
% G24 = [cos(sita12) d*sin(sita12);
%        sin(sita24) d*cos(sita24)];
% F4 = [-u1(1)*cos(mega12);0];
% vw4 = inv(G24)*(p4 - F4);
% %%%%%
% 
% %%%%
% x5=2.5;
% y5 =2;
% theta5 = 2*pi/3;
% 
% L35_x=x3-x5-d*cos(theta5);
% L35_y=y3-y5-d*sin(theta5);
% 
% L35=sqrt(L35_x^2+L35_y^2);
% sita13 = theta1 - theta3 + mega13;
% sita35 = theta5 - theta3;
% 
% p5 = [k(1)*(target(3) - L13);
%       5*(0.09 - L35)];
% G35 = [cos(sita13) d*sin(sita13);
%        sin(sita35) d*cos(sita35)];
% F5 = [-u1(1)*cos(mega13);0];
% vw5 = inv(G35)*(p5 - F5);
% %%%%%
% 
% if L24<0.1
%     y = [vw4(1);vw4(2);u(3);u(4)];
% elseif L35 < 0.09
%         y = [u(1);u(2);vw5(1);vw5(2)];
% elseif (L35 < 0.1)&&(L24<0.1)
%         y = [vw4(1);vw4(2);vw5(1);vw5(2)];
% else
%     y=u;
% end

== matlab function formationControl/MATLAB Function ==
  data: delta input; y output; theta0_present input; k input; vw input; vw1 output
function [y,vw1] = fcn(delta,theta0_present,k,vw)

%#codegen
A=[cos(theta0_present)   sin(theta0_present) 0;
    -sin(theta0_present) cos(theta0_present) 0;
    0                    0                    1];
e=A*delta;
V_c=[vw(1)*cos(e(3))+k(1)*e(1);
    vw(2)+k(2)*vw(1)*e(2)+k(3)*vw(1)*sin(e(3))];
limit=5;
if abs(V_c(1)) >limit
    V_c(1) =(V_c(1)/abs(V_c(1)))*limit;
end
if abs(V_c(2))>limit
    V_c(2) =(V_c(2)/abs(V_c(2)))*limit;
end

Matrix=[cos(theta0_present) 0;
        sin(theta0_present) 0;
        0                   1];
u=Matrix*V_c;
y = u;
vw1=V_c;

== matlab function formationControl/MATLAB Function2 ==
  data: x1 input; y output; y1 input; xr input; yr input
function y = fcn(x1,y1,xr,yr)
%#codegen
x_delta=xr-x1;
y_delta=yr-y1;

y=atan2(y_delta,x_delta);
if y<0 %khi mega <0 se xay ra hien tuong xoay tron
    k13=fix(-y/(2*pi));
    y = 2*(k13+1)*pi +y;
end
if y>(2*pi) %khi mega <0 se xay ra hien tuong xoay tron
    k13=fix(y/(2*pi));
    y = y-2*(k13+1)*pi;
end
% if y<0
%     k1=fix(-y/(2*pi));
%     y = 2*(k1+1)*pi +y;
% end

== matlab function formationControl/MATLAB Function3 ==
  data: parameter input; y output; theta2_present input
function y = fcn(parameter,theta2_present)
%#codegen
d=0.09;
Matrix=[cos(theta2_present) -d*sin(theta2_present);
        sin(theta2_present) d*cos(theta2_present);
        0                   1];
% Matrix=[cos(theta2_present) 0;
%         sin(theta2_present) 0;
%         0                   1];
u=Matrix*parameter;
y = u;

== matlab function formationControl/MATLAB Function4 ==
  data: parameter input; y3 output; theta3_present input
function y3 = fcn(parameter,theta3_present)
%#codegen
d=0.09;
Matrix=[cos(theta3_present) -d*sin(theta3_present);
        sin(theta3_present) d*cos(theta3_present);
        0                   1];
% Matrix=[cos(theta3_present) 0;
%         sin(theta3_present) 0;
%         0                   1];
u=Matrix*parameter;
y3 = u;

== matlab function formationControl/MATLAB Function5 ==
  data: x output; t input; y output; theta output
function [x,y,theta] = fcn(t)
%#codegen
x = (t^3)/1000;
y = t;

theta = pi/2;

== matlab function formationControl/MATLAB Function6 ==
  data: x1 input; target output; y1 input; theta1 input; x2 input; y2 input; theta2 input; x3 input; y3 input; theta3 input
function target = fcn(x1,y1,theta1,x2,y2,theta2,x3,y3,theta3)
%#codegen
d=0.09;
% 
% L12_x=x1-x2-d*cos(theta1);
% L12_y=y1-y2-d*sin(theta1);
% L13_x=x1-x3-d*cos(theta1);
% L13_y=y1-y3-d*sin(theta1);
% L23_x=x2-x3-d*cos(theta2);
% L23_y=y2-y3-d*sin(theta2);
L12_x=x1-x2-d*cos(theta2);
L12_y=y1-y2-d*sin(theta2);
L13_x=x1-x3-d*cos(theta3);
L13_y=y1-y3-d*sin(theta3);
L23_x=x2-x3-d*cos(theta3);
L23_y=y2-y3-d*sin(theta3);

L12=sqrt(L12_x^2+L12_y^2);
L13=sqrt(L13_x^2+L13_y^2);
L23=sqrt(L23_x^2+L23_y^2);

mega12=atan2(L12_y,L12_x)-theta1+pi;
if mega12<0
    k12=fix(-mega12/(2*pi));
    mega12 = 2*(k12+1)*pi +mega12;
end
mega13 = atan2(L13_y,L13_x)-theta1+pi;
if mega13<0 %khi mega <0 se xay ra hien tuong xoay tron
    k13=fix(-mega13/(2*pi));
    mega13 = 2*(k13+1)*pi +mega13;
end
% mega23=atan2(L23_y,L23_x)-theta2+pi;
% if mega23<0 %khi mega <0 se xay ra hien tuong xoay tron
%     k23=fix(-mega23/(2*pi));
%     mega23 = 2*(k23+1)*pi +mega23;
% end
target=[L12;mega12;L13;mega13];
